simulink model "RC_Circute"  (R2023a)
settings: Solver=FixedStepAuto  StartTime=0.0  StopTime=10.0  MaxStep=1e-3  RelTol=1e-3
values from neighbouring files (symbols this model uses):
  C = 1e-6    (= 1e-06)    [RC_sim.m]
  R = 1    [RC_sim.m]
settings Model: Creator=Mohamed Ezzelrgal  LastModifiedBy=Mohamed Ezzelrgal
settings OptimizationCC: DefaultParameterBehavior=Inlined  UseDivisionForNetSlopeComputation=on  GainParamInheritBuiltInType=on  UseFloatMulNetSlope=on  InlineInvariantSignals=on  PassReuseOutputArgsAs=Individual arguments  ZeroExternalMemoryAtStartup=off  ZeroInternalMemoryAtStartup=off  NoFixptDivByZeroProtection=on  EfficientFloat2IntCast=on  LifeSpan=1  OptimizeBlockOrder=speed  DifferentSizesBufferReuse=on  EfficientTunableParamExpr=on
settings DebuggingCC: ParameterTunabilityLossMsg=error
settings HardwareCC: ProdBitPerInt=16  ProdBitPerPointer=16  ProdBitPerSizeT=16  ProdBitPerPtrDiffT=16  ProdLargestAtomicFloat=None  ProdWordSize=8  ProdLongLongMode=on  ProdHWDeviceType=Atmel->AVR
settings SFSimCC: MATLABDynamicMemAlloc=off
settings RTWCC: Description=Embedded Coder  SystemTargetFile=ert.tlc  TemplateMakefile=ert_default_tmf
settings CodeAppCC: ForceParamTrailComments=on  IgnoreCustomStorageClasses=off  OperatorAnnotations=on  SimulinkDataObjDesc=on  SFDataObjDesc=on  CustomSymbolStrGlobalVar=rt$N$M  CustomSymbolStrType=$N$M  CustomSymbolStrFcn=$N$M$F  CustomSymbolStrMacro=$N$M  InsertBlockDesc=on
settings ERTTargetCC: TargetLangStandard=C99 (ISO)  GenerateSampleERTMain=on  IncludeMdlTerminateFcn=off  CombineSignalStateStructs=on  SupportComplex=off  SupportContinuousTime=on  InlinedParameterPlacement=NonHierarchical  ERTCustomFileTemplate=example_file_process.tlc  ERTFilePackagingFormat=CompactWithDataFile

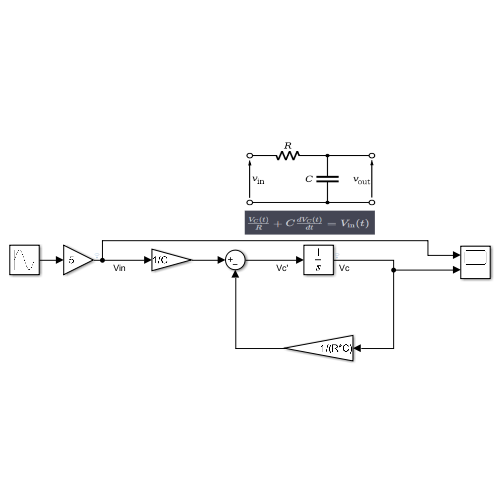
[thumbnail: Simulink's stored preview of the top-level diagram]
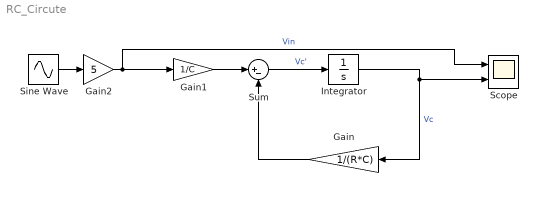
== system RC_Circute ==
  Gain : Gain  Gain=1/(R*C)
  Gain1 : Gain  Gain=1/C
  Gain2 : Gain  Gain=5
  Integrator : Integrator  InitialCondition=1
  Scope : Scope  NumInputPorts=2
  Sine Wave : Sin  Frequency=2*pi  SampleTime=0
  Sum : Sum  Inputs=|+-
  wires:
  Sum/1 -> Integrator/1  "Vc'"
  Integrator/1 -> Scope/2, Gain/1  "Vc"
  Sine Wave/1 -> Gain2/1
  Gain/1 -> Sum/2
  Gain2/1 -> Scope/1, Gain1/1  "Vin"
  Gain1/1 -> Sum/1
